simulink model "updated_seven_dof_vehicle_model"  (R2025b)
settings: Solver=ode23tb  StartTime=0.0  StopTime=37  MaxStep=0.001  RelTol=1e-3
model workspace (MAT data in the model file):
  init_r = 0
  init_vx = 0
  init_vy = 0
values from neighbouring files (symbols this model uses):
  Par =     [New_Load_data for_7DOF.mat]
  TireData =     [New_Load_data for_7DOF.mat]
libraries: simulink x3
(part 2 of 2)

== matlab function updated_seven_dof_vehicle_model/Steering Kinematics/Steering Kinematics ==
  data: Steer_Input input; Ackermann_Pct input; Steer_FL output; Steer_FR output; Par parameter
function [Steer_FL, Steer_FR] = fcn(Steer_Input, Ackermann_Pct, Par)
%#codegen

    % 1. Constants
    L = Par.WB;      % Wheelbase
    half_T = Par.TW / 2; % Half Track Width

    % 2. Safety Clamp (Prevent tan(90) singularity)
    delta = min(max(Steer_Input, -1.5), 1.5); 
    
    % 3. Calculate "Pure Ackermann" Angles
    % Ideally, inner wheel turns sharper than outer wheel.
    tan_d = tan(delta);
    
    % FL (Left): Denom depends on sign of turn.
    % If turning Left (+), Denom shrinks (Sharper).
    FL_Ack = atan( (L * tan_d) / (L - half_T * tan_d) );
    
    % FR (Right): 
    % If turning Left (+), Denom grows (Shallower).
    FR_Ack = atan( (L * tan_d) / (L + half_T * tan_d) );
    
    % 4. Calculate "Parallel" Angles
    % Both wheels exactly match the center input
    FL_Par = delta;
    FR_Par = delta;
    
    % 5. Linear Blend based on Percentage
    % Formula: Final = Parallel + (Ackermann - Parallel) * Percent
    Steer_FL = FL_Par + (FL_Ack - FL_Par) * Ackermann_Pct;
    Steer_FR = FR_Par + (FR_Ack - FR_Par) * Ackermann_Pct;

end

== matlab function updated_seven_dof_vehicle_model/Wheel Dynamics/MATLAB Function ==
  data: T_in input; Omega_dot output; Fx_rr input; Fx_tire input; Omega input; Par parameter
function Omega_dot = fcn(T_in, Fx_rr,Fx_tire, Omega, Par)
%#codegen

    % 1. Constants
    R = Par.R0;
    Iw = Par.I_wheel;

    % 2. Separate Drive and Brake components

    T_drive = max(T_in, 0); 
    
    % T_brake is the magnitude of the negative part of T_in
    T_brake_mag = abs(min(T_in, 0));
    

    Rotation_Dir = tanh(10 * Omega);

    % 4. Calculate Net Torque
    T_tire_reaction = abs(Fx_rr .* R);
    T_tire = Fx_tire .*R;
    T_damping = 0.1*Omega;
    T_net = T_drive - (T_brake_mag .* Rotation_Dir) - (T_tire_reaction.*Rotation_Dir) -T_tire - T_damping;

    % 5. Compute Angular Acceleration
    Omega_dot = T_net ./ Iw;

end
